simulink model "EASY_PASS"  (R2019b)
settings: Solver=VariableStepAuto  StartTime=0.0  StopTime=10.0  RelTol=1e-3
undefined symbols (not defined in the file or in its folder): m, n
settings Model: Creator=Εμμανουήλ  LastModifiedBy=Εμμανουήλ

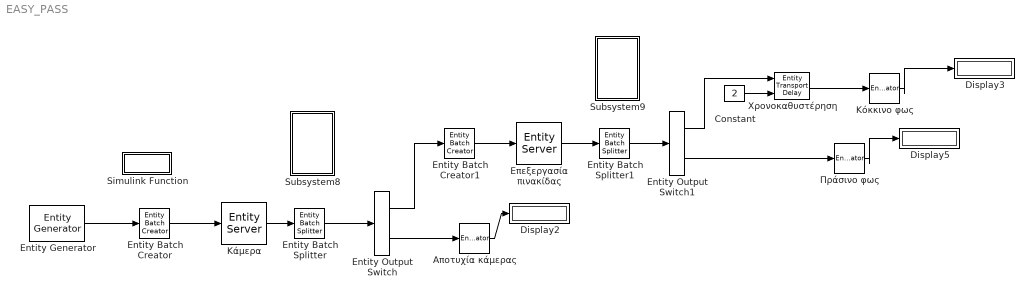
== system EASY_PASS ==
  Constant : Constant  Value=2
  Display2 : Display
  Display3 : Display
  Display5 : Display
  Entity Output Switch : EntityOutputSwitch  InputPortMessageModes=m  OutputPortMessageModes=m,m  SwitchingCriterion=From attribute  SwitchAttributeName=car
  Entity Output Switch1 : EntityOutputSwitch  InputPortMessageModes=m  OutputPortMessageModes=m,m  SwitchingCriterion=From attribute  SwitchAttributeName=result
  Entity Batch Creator : EntityBatchCreator  InputPortMessageModes=m  OutputPortMessageModes=m  NumberOfEntitiesInBatch=9
      settings: OutputPortMap=o4
  Entity Batch Creator1 : EntityBatchCreator  InputPortMessageModes=m  OutputPortMessageModes=m  NumberOfEntitiesInBatch=2  EntityTypeName=B  InputEntityName=b  EntryAction=entity.result = ismember(entity.namber,G)+1;
      settings: OutputPortMap=o4
  Entity Batch Splitter : EntityBatchSplitter  InputPortMessageModes=m  OutputPortMessageModes=m  ExitAction=|
      | if (entity.car==2)
      |     Failure(entity.car)
      | else 
      |     Success(entity.car)
      | end
      settings: OutputPortMap=o4
  Entity Batch Splitter1 : EntityBatchSplitter  InputPortMessageModes=m  OutputPortMessageModes=m  ExitAction=|
      | if (entity.result==1)
      |    Red(entity.namber)
      | elseif (entity.result==2)
      |     Green(entity.namber)
      | end
      settings: OutputPortMap=o4
  Entity Generator : EntityGenerator  OutputPortMessageModes=m  Period=10  IntergenerationTimeAction=dt = DT;  GenerateAction=|  AttributeName=namber|car|result  AttributeInitialValue=1|1|1  EntityType=Structured  EntityTypeName=Vehicles
      | entity.namber = randi([1000 9999]);
      | entity.car = f();
  Simulink Function : Subsystem  TreatAsAtomicUnit=on
  Subsystem8 : Subsystem
  Subsystem9 : Subsystem
  Αποτυχία κάμερας : EntityTerminator  InputPortMessageModes=m  NumberEntitiesArrived=on
      settings: OutputPortMap=o0
  Επεξεργασία πινακίδας : EntityServer  InputPortMessageModes=m  OutputPortMessageModes=m  Capacity=1  ServiceTimeValue=.1  ExitAction=|
      | entity.b(1).result=1;
      | entity.b(2).result=2;
  Κάμερα : EntityServer  InputPortMessageModes=m  OutputPortMessageModes=m  Capacity=1  ServiceTimeValue=.2  EntryAction=entity.batch(f()).car = f();
  Κόκκινο φως : EntityTerminator  InputPortMessageModes=m  NumberEntitiesArrived=on
      settings: OutputPortMap=o0
  "Πράσινο φως " : EntityTerminator  InputPortMessageModes=m  NumberEntitiesArrived=on
      settings: OutputPortMap=o0
  Χρονοκαθυστέρηση : EntityTransportDelay  InputPortMessageModes=m,n  OutputPortMessageModes=m
  wires:
  Entity Output Switch1/1 -> Χρονοκαθυστέρηση/1
  Κόκκινο φως/1 -> Display3/1
  "Πράσινο φως "/1 -> Display5/1
  Αποτυχία κάμερας/1 -> Display2/1
  Constant/1 -> Χρονοκαθυστέρηση/2
  Entity Output Switch/2 -> Αποτυχία κάμερας/1
  Χρονοκαθυστέρηση/1 -> Κόκκινο φως/1
  Entity Batch Splitter1/1 -> Entity Output Switch1/1
  Entity Output Switch/1 -> Entity Batch Creator1/1
  Επεξεργασία πινακίδας/1 -> Entity Batch Splitter1/1
  Entity Batch Splitter/1 -> Entity Output Switch/1
  Entity Output Switch1/2 -> "Πράσινο φως "/1
  Entity Batch Creator/1 -> Κάμερα/1
  Κάμερα/1 -> Entity Batch Splitter/1
  Entity Batch Creator1/1 -> Επεξεργασία πινακίδας/1
  Entity Generator/1 -> Entity Batch Creator/1

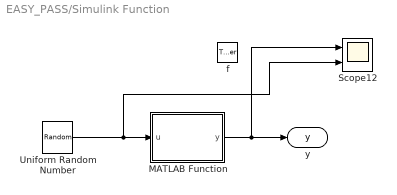
== system EASY_PASS/Simulink Function ==
  f : TriggerPort  TriggerType=function-call  IsSimulinkFunction=on  FunctionName=f  FunctionVisibility=scoped  VariantControl=(inherit)
  MATLAB Function : MATLAB Function  TreatAsAtomicUnit=on
  Scope12 : Scope  NumInputPorts=2
  Uniform Random Number : UniformRandomNumber  Minimum=0
  y : ArgOut  DisableCoverage=on  ArgumentName=y
  wires:
  Uniform Random Number/1 -> Scope12/2, MATLAB Function/1(u)
  MATLAB Function/1(y) -> Scope12/1, y/1

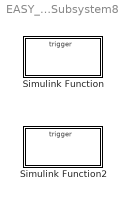
== system EASY_PASS/Subsystem8 ==
  Simulink Function : Subsystem  TreatAsAtomicUnit=on
  Simulink Function2 : Subsystem  TreatAsAtomicUnit=on

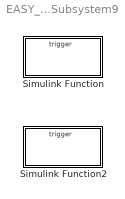
== system EASY_PASS/Subsystem9 ==
  Simulink Function : Subsystem  TreatAsAtomicUnit=on
  Simulink Function2 : Subsystem  TreatAsAtomicUnit=on

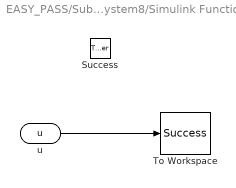
== system EASY_PASS/Subsystem8/Simulink Function ==
  Success : TriggerPort  TriggerType=function-call  IsSimulinkFunction=on  FunctionName=Success  VariantControl=(inherit)
  To Workspace : ToWorkspace  VariableName=Success  SampleTime=-1
      settings: Save2DSignal=2-D array (concatenate along first dimension)
  u : ArgIn  DisableCoverage=on  ArgumentName=u
  wires:
  u/1 -> To Workspace/1

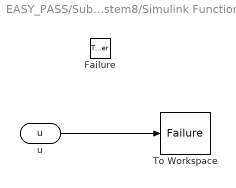
== system EASY_PASS/Subsystem8/Simulink Function2 ==
  Failure : TriggerPort  TriggerType=function-call  IsSimulinkFunction=on  FunctionName=Failure  VariantControl=(inherit)
  To Workspace : ToWorkspace  VariableName=Failure  SampleTime=-1
      settings: Save2DSignal=2-D array (concatenate along first dimension)
  u : ArgIn  DisableCoverage=on  ArgumentName=u
  wires:
  u/1 -> To Workspace/1

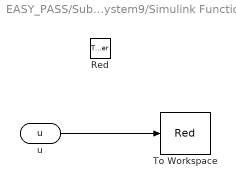
== system EASY_PASS/Subsystem9/Simulink Function ==
  Red : TriggerPort  TriggerType=function-call  IsSimulinkFunction=on  FunctionName=Red  VariantControl=(inherit)
  To Workspace : ToWorkspace  VariableName=Red  SampleTime=-1
      settings: Save2DSignal=2-D array (concatenate along first dimension)
  u : ArgIn  DisableCoverage=on  ArgumentName=u
  wires:
  u/1 -> To Workspace/1

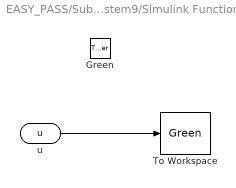
== system EASY_PASS/Subsystem9/Simulink Function2 ==
  Green : TriggerPort  TriggerType=function-call  IsSimulinkFunction=on  FunctionName=Green  VariantControl=(inherit)
  To Workspace : ToWorkspace  VariableName=Green  SampleTime=-1
      settings: Save2DSignal=2-D array (concatenate along first dimension)
  u : ArgIn  DisableCoverage=on  ArgumentName=u
  wires:
  u/1 -> To Workspace/1

== matlab function EASY_PASS/Simulink Function/MATLAB Function ==
  data: u input; y output
function y = fcn(u)
if ( u <=.2 )
    y=2; 
else
    y=1;
end
